simulink model "DoubleIntegratorNMPCSimulink"  (R2018a)
settings: Solver=ode1  StartTime=0.0  StopTime=6  FixedStep=tstep  RelTol=1e-3
InitFcn:
  | initSim;
StopFcn:
  | plotSimSolution;
values from neighbouring files (symbols this model uses):
  tstep = 0.01    [initSim.m]
undefined symbols (not defined in the file or in its folder): m, problem
settings Model: SimulationMode=accelerator  Creator=yn15  LastModifiedBy=yesid
settings OptimizationCC: LifeSpan=inf
settings DebuggingCC: SFUnexpectedBacktrackingDiag=warning  SFNoUnconditionalDefaultTransitionDiag=warning  SFExecutionAtInitializationDiag=none
settings CodeAppCC: StateflowObjectComments=on
settings GRTTargetCC: TargetLangStandard=C89/C90 (ANSI)
settings ConfigComp: CovMetricSettings=dw  CovHtmlReporting=on  CovSaveCumulativeToWorkspaceVar=on  CovSaveSingleToWorkspaceVar=on  CovExternalEMLEnable=off

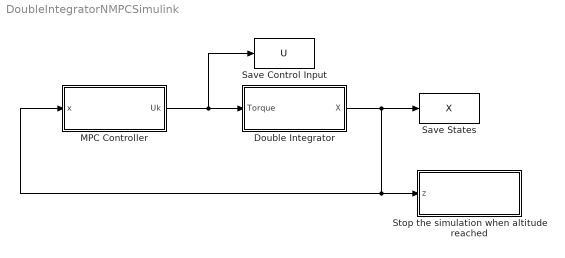
== system DoubleIntegratorNMPCSimulink ==
  Double Integrator : Subsystem
  "MPC Controller " : Subsystem
  Save Control Input : ToWorkspace  VariableName=U  SampleTime=-1
      settings: Save2DSignal=2-D array (concatenate along first dimension)
  Save States : ToWorkspace  VariableName=X  SampleTime=-1
  "Stop the simulation when altitude reached " : Subsystem
  wires:
  "MPC Controller "/1(Uk) -> Save Control Input/1, Double Integrator/1(Torque)
  Double Integrator/1(X) -> Save States/1, "Stop the simulation when altitude reached "/1(z), "MPC Controller "/1(x)

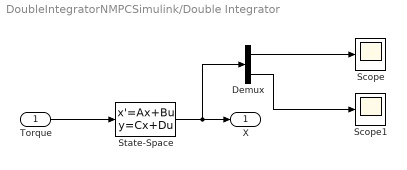
== system DoubleIntegratorNMPCSimulink/Double Integrator ==
  Torque : Inport
  Demux : Demux  Outputs=2
  Scope : Scope
  Scope1 : Scope
  State-Space : StateSpace  A=[0 1;0 0]  B=[0;1]  C=[1 0;0 1]  D=[0;0]  InitialCondition=0
  X : Outport
  wires:
  State-Space/1 -> Demux/1, X/1
  Demux/1 -> Scope/1
  Demux/2 -> Scope1/1
  Torque/1 -> State-Space/1

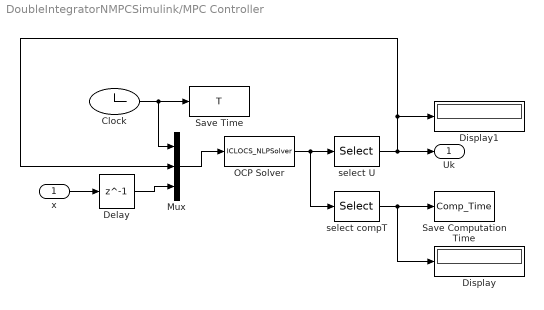
== system DoubleIntegratorNMPCSimulink/MPC Controller  ==
  x : Inport
  Clock : Clock
  Delay : Delay  DelayLength=1  InitialCondition=[problem.states.x0]
  Display : Display
  Display1 : Display
  Mux : Mux  Inputs=3
  OCP Solver : MATLABFcn  MATLABFcn=ICLOCS_NLPSolver  OutputDimensions=m+2
  "Save Computation Time " : ToWorkspace  VariableName=Comp_Time  SampleTime=tstep
      settings: Save2DSignal=2-D array (concatenate along first dimension)
  Save Time : ToWorkspace  VariableName=T  SampleTime=-1
      settings: Save2DSignal=2-D array (concatenate along first dimension)
  select U : Selector  IndexOptions=Index vector (dialog)  Indices=3:m+2  OutputSizes=1
  select compT : Selector  IndexOptions=Index vector (dialog)  Indices=2  OutputSizes=1
  Uk : Outport
  wires:
  select U/1 -> Mux/2, Display1/1, Uk/1
  x/1 -> Delay/1
  OCP Solver/1 -> select compT/1, select U/1
  Clock/1 -> Save Time/1, Mux/1
  Mux/1 -> OCP Solver/1
  select compT/1 -> Display/1, "Save Computation Time "/1
  Delay/1 -> Mux/3

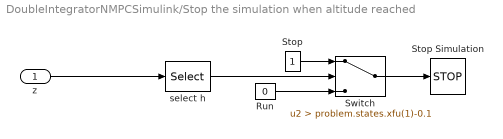
== system DoubleIntegratorNMPCSimulink/Stop the simulation when altitude reached  ==
  z : Inport
  Run : Constant  Value=0
  Stop : Constant
  Stop Simulation : Stop
  Switch : Switch  Criteria=u2 > Threshold  Threshold=problem.states.xfu(1)-0.1
  select h : Selector  IndexOptions=Index vector (dialog)  Indices=1  OutputSizes=1
  wires:
  Switch/1 -> Stop Simulation/1
  z/1 -> select h/1
  Stop/1 -> Switch/1
  Run/1 -> Switch/3
  select h/1 -> Switch/2
